simulink model "adrc1"  (Simulink 7.6)
settings: Solver=ode3  StartTime=0.0  StopTime=100  FixedStep=0.1  RelTol=1e-3
settings Model: Creator=Administrator  LastModifiedBy=Administrator
settings OptimizationCC: InitFltsAndDblsToZero=on
settings DebuggingCC: AlgebraicLoopMsg=none  SaveWithParameterizedLinksMsg=none  SignalResolutionControl=TryResolveAllWithWarning  SolverPrmCheckMsg=none  MultiTaskDSMMsg=warning  MultiTaskCondExecSysMsg=none  StrictBusMsg=None
settings RTWCC: IncludeERTFirstTime=on
settings GRTTargetCC: TargetFcnLib=ansi_tfl_tmw.mat

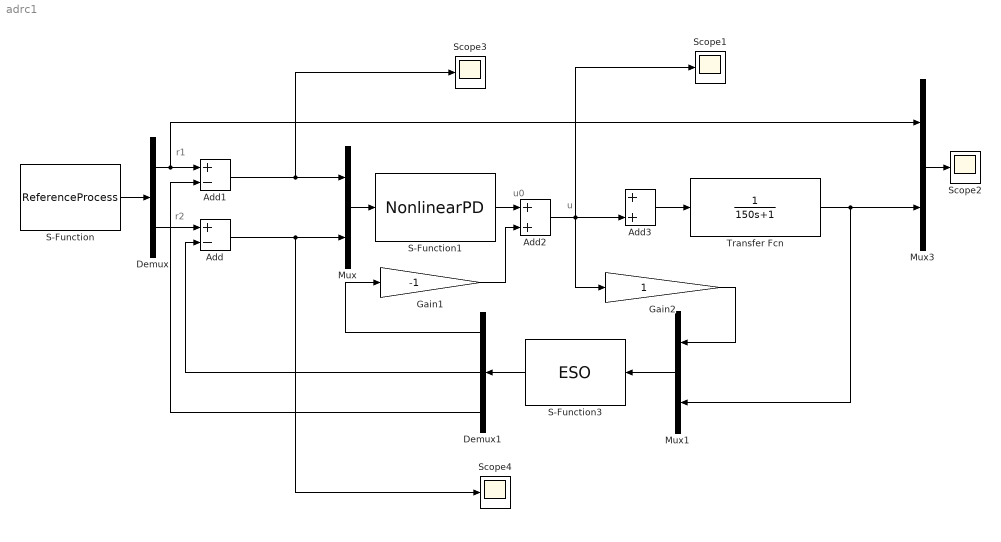
== system adrc1 ==
  note: u0
  note: r1
  note: r2
  note: u
  Add : Sum  Inputs=+-
  Add1 : Sum  Inputs=+-
  Add2 : Sum
  Add3 : Sum
  Demux : Demux  Outputs=2
  Demux1 : Demux  Outputs=3
  Gain1 : Gain  Gain=-1
  Gain2 : Gain
  Mux : Mux  Inputs=2
  Mux1 : Mux  Inputs=2
  Mux3 : Mux  Inputs=2
  S-Function : S-Function  FunctionName=ReferenceProcess  Parameters=SetPoint, RisingTime,SampleTime  EnableBusSupport=off  mask{SetPoint=5, RisingTime=50, SampleTime=0.1}
  S-Function1 : S-Function  FunctionName=NonlinearPD  Parameters=Beta1,Beta2,Delta,A1,A2,SampleTime  EnableBusSupport=off  mask{Beta1=3000, Beta2=2000, Delta=0.1, A1=0.25, A2=0.75, SampleTime=0.1}
      mask prompts: Beta1 "Proportion Coefficient"; Beta2 "Derivation Coefficient"; A1 "Proportion Power"; A2 "Derivation Power"; SampleTime "Sample Time"
  S-Function3 : S-Function  FunctionName=ESO  Parameters=SampleTime,Delta,Beta1,Beta2,Beta3  EnableBusSupport=off  mask{Delta=0.1, Beta1=100, Beta2=65, Beta3=85, SampleTime=0.1}
      mask prompts: Delta "Linear Region"; Beta1 "Observer Coefficient 1"; Beta2 "Observer Coefficient 2"; Beta3 "Observer Coefficient 3"; SampleTime "Sample Time"
  Scope{1..4} (4 alike) : Scope
      Scope1 settings: TimeRange=3.16679535927733e-007  YMin=0.996252  YMax=0.99644
      Scope2 settings: TimeRange=24  YMin=0.852020202020202  YMax=0.859090909090909  SaveName=ScopeData10
      Scope3 settings: TimeRange=3.16679535927733e-007  YMin=0.9962515155865817  YMax=0.9964397232263716
      Scope4 settings: TimeRange=3.16679535927733e-007  YMin=0.996252  YMax=0.99644  SaveName=ScopeData2
  Transfer Fcn : TransferFcn  Numerator=1  Denominator=[150 1]
  wires:
  S-Function/1 -> Demux/1
  Demux/2 -> Add/1
  Demux/1 -> Add1/1, Mux3/1
  S-Function3/1 -> Demux1/1
  Demux1/3 -> Add1/2
  Demux1/2 -> Add/2
  Add1/1 -> Mux/1, Scope3/1
  Add/1 -> Mux/2, Scope4/1
  Mux/1 -> S-Function1/1
  Add2/1 -> Gain2/1, Add3/2, Scope1/1
  Transfer Fcn/1 -> Mux1/2, Mux3/2
  Mux1/1 -> S-Function3/1
  Demux1/1 -> Gain1/1
  Gain1/1 -> Add2/2
  S-Function1/1 -> Add2/1
  Gain2/1 -> Mux1/1
  Mux3/1 -> Scope2/1
  Add3/1 -> Transfer Fcn/1
